simulink library "ReceiveFromPDB"  (R2016b)
settings: Solver=VariableStepAuto  StartTime=0.0  StopTime=10.0  RelTol=1e-3
settings Model: Creator=Nathan  LastModifiedBy=march

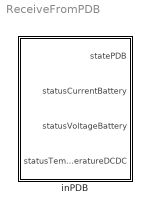
== system ReceiveFromPDB ==
  inPDB : Subsystem

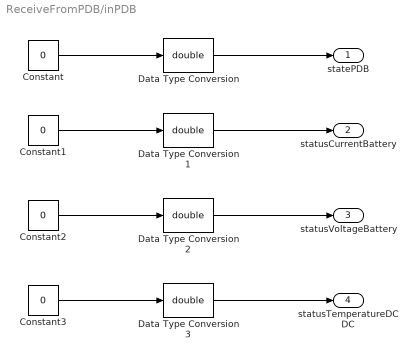
== system ReceiveFromPDB/inPDB ==
  Constant{,1..3} (4 alike) : Constant  Value=0
  Data Type Conversion{,1..3} (4 alike) : DataTypeConversion  OutDataTypeStr=double
  statePDB : Outport
  statusCurrentBattery : Outport  Port=2
  statusVoltageBattery : Outport  Port=3
  statusTemperatureDCDC : Outport  Port=4
  wires:
  Constant3/1 -> Data Type Conversion3/1
  Constant2/1 -> Data Type Conversion2/1
  Constant1/1 -> Data Type Conversion1/1
  Constant/1 -> Data Type Conversion/1
  Data Type Conversion/1 -> statePDB/1
  Data Type Conversion1/1 -> statusCurrentBattery/1
  Data Type Conversion2/1 -> statusVoltageBattery/1
  Data Type Conversion3/1 -> statusTemperatureDCDC/1
